simulink model "EV_Modeling_old"  (R2024b)
settings: Solver=FixedStepAuto  StartTime=0.0  StopTime=10382  FixedStep=0.1  RelTol=1e-3
values from neighbouring files (symbols this model uses):
  battery_SOC_SOC = battery_SOC(:,1)    [EV_Truck.m]    (also in simulink.m)
  battery_SOC_voltage = battery_SOC(:,2)    [EV_Truck.m]    (also in simulink.m)
  drag_coefficient_FV1 = table2array(drag_coefficient(:,3))    [simulink.m]
  drag_coefficient_FV2 = table2array(drag_coefficient(:,4))    [simulink.m]
  drag_coefficient_input = table2array(drag_coefficient(:,1))    [simulink.m]
  drag_coefficient_LV = table2array(drag_coefficient(:,2))    [simulink.m]
  electric_consumption_ressistancce = electric_consumption(:,2)    [EV_Truck.m]    (also in simulink.m)
  electric_consumption_voltage = electric_consumption(:,1)    [EV_Truck.m]    (also in simulink.m)
  motor_efficiency_efficiency = table2array(motor_efficiency(2:height(motor_efficiency),2:width(motor_efficiency)))    [EV_Truck.m]    (also in simulink.m)
  motor_efficiency_RPM = table2array(motor_efficiency(2:height(motor_efficiency),1))    [EV_Truck.m]    (also in simulink.m)
  motor_efficiency_torque = transpose(motor_efficiency_torque)    [EV_Truck.m]    (also in simulink.m)
  motor_RPM_torque = table2array(motor_torque(1:14,1))    [EV_Truck.m]    (also in simulink.m)
  motor_torque_RPM = table2array(motor_torque(1:14,2))    [EV_Truck.m]    (also in simulink.m)
undefined symbols (not defined in the file or in its folder): battery_builder_rtmsupport, battery_sli_rtmsupport, C1_mat, C2_mat, c_sqrt, DiscIntNeverNeededParam, dV0_mat, gcbh, n, Wc, Wm, x0
libraries: simulink x87, packLibrary_lib x30, nesl_utility x6, fl_lib x6, simulink_extras x3, mpcadaslib x2, slpidlib x1
(part 1 of 12)
settings Model: Creator=Administrator  LastModifiedBy=avees
settings SolverCC: AlgebraicLoopSolver=TrustRegion
settings DataIOCC: ExternalInput=EV_ModelingScenario.getElement('Input')  LoadExternalInput=on
settings DebuggingCC: UnconnectedInputMsg=warning  UnconnectedOutputMsg=warning  UnconnectedLineMsg=warning
settings ModelReferenceCC: EnableRefExpFcnMdlSchedulingChecks=on
settings RTWCC: GPUComputeCapability=3.5  DLArmComputeVersion=19.05

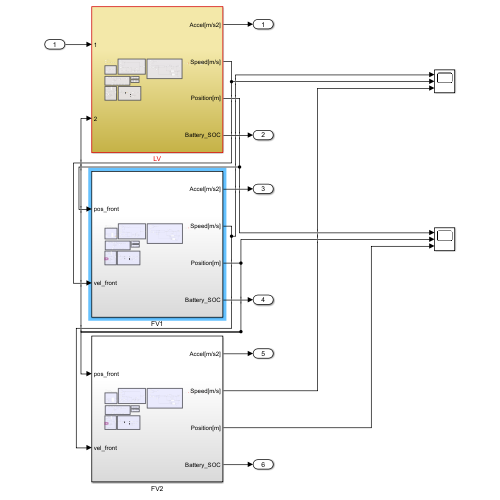
[thumbnail: Simulink's stored preview of the top-level diagram]
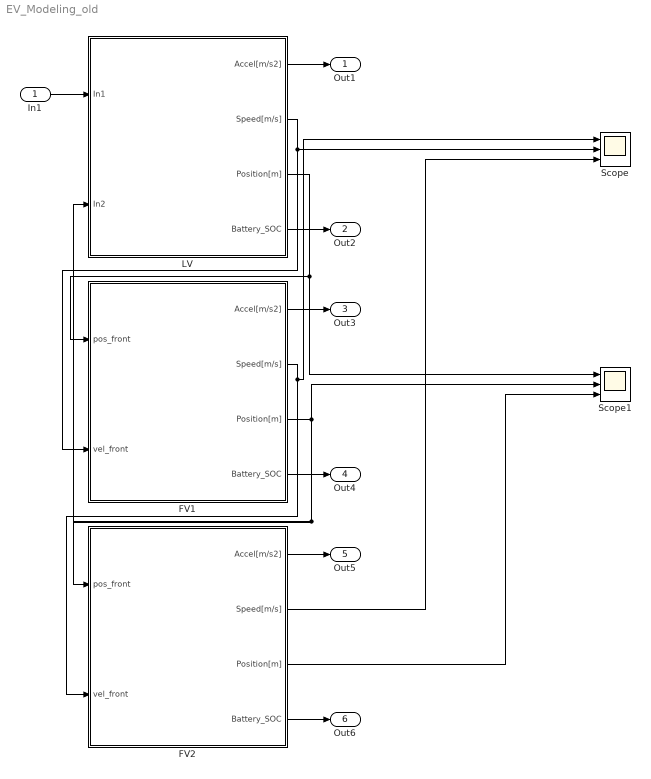
== system EV_Modeling_old ==
  In1 : Inport
  FV1 : Subsystem
  FV2 : Subsystem
  LV : Subsystem
  Scope : Scope  NumInputPorts=3
  Scope1 : Scope  NumInputPorts=3
  Out1 : Outport
  Out2 : Outport  Port=2
  Out3 : Outport  Port=3
  Out4 : Outport  Port=4
  Out5 : Outport  Port=5
  Out6 : Outport  Port=6
  wires:
  In1/1 -> LV/1(In1)
  LV/3(Position[m]) -> Scope1/1, FV1/1(pos_front)
  LV/2(Speed[m/s]) -> FV1/2(vel_front), Scope/2
  FV1/2(Speed[m/s]) -> FV2/2(vel_front), Scope/1
  FV1/3(Position[m]) -> LV/2(In2), FV2/1(pos_front), Scope1/2
  LV/1(Accel[m/s2]) -> Out1/1
  LV/4(Battery_SOC) -> Out2/1
  FV1/1(Accel[m/s2]) -> Out3/1
  FV1/4(Battery_SOC) -> Out4/1
  FV2/1(Accel[m/s2]) -> Out5/1
  FV2/2(Speed[m/s]) -> Scope/3
  FV2/3(Position[m]) -> Scope1/3
  FV2/4(Battery_SOC) -> Out6/1

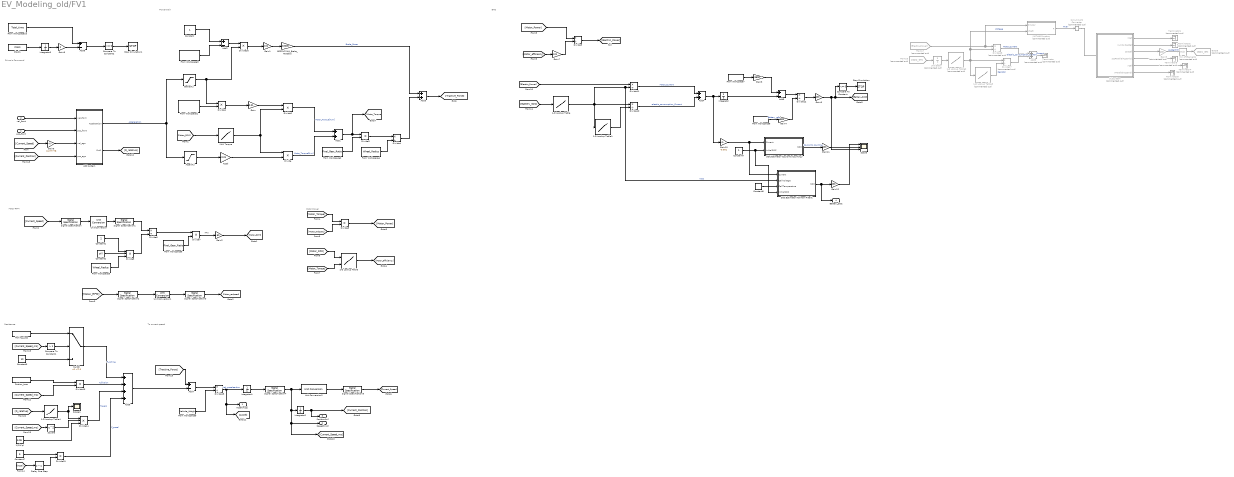
== system EV_Modeling_old/FV1 ==
  note: BMS
  note: To current speed
  note: Motor Power
  note: Power train
  note: Driver's Command
  note: RPS
  note: Motor RPM
  note: Resistance
  pos_front : Inport
  vel_front : Inport  Port=2
  1-D Lookup Table : Lookup_n-D  NumberOfTableDimensions=1  BreakpointsForDimension1=battery_SOC_SOC  Table=battery_SOC_voltage  InternalRulePriority=Speed  RndMeth=Simplest
  1-D Lookup Table1 : Lookup_n-D  NumberOfTableDimensions=1  BreakpointsForDimension1=electric_consumption_voltage  Table=electric_consumption_ressistancce  InternalRulePriority=Speed  RndMeth=Simplest
  1-D Lookup Table2 : Lookup_n-D  Commented=on  NumberOfTableDimensions=1  BreakpointsForDimension1=battery_SOC_SOC  Table=battery_SOC_voltage  InternalRulePriority=Speed  RndMeth=Simplest
  1-D Lookup Table3 : Lookup_n-D  Commented=on  NumberOfTableDimensions=1  BreakpointsForDimension1=electric_consumption_voltage  Table=electric_consumption_ressistancce  InternalRulePriority=Speed  RndMeth=Simplest
  1-D Lookup Table4 : Lookup_n-D  NumberOfTableDimensions=1  BreakpointsForDimension1=drag_coefficient_input  Table=drag_coefficient_FV1  InternalRulePriority=Speed  RndMeth=Simplest
  1/2(A*p) : Constant  Value=5.06
  2-D Lookup Table : Lookup_n-D  BreakpointsForDimension1=motor_efficiency_RPM  BreakpointsForDimension2=motor_efficiency_torque  Table=motor_efficiency_efficiency  InternalRulePriority=Speed  RndMeth=Simplest
      settings: InputPortMap=u0,u1
  ACC system : Subsystem
  Accel : Gain  Gain=0.01
  Accel[%] : Saturate  UpperLimit=100  LowerLimit=0
  Add1 : Sum
  Add{2,5,7..8} (4 alike) : Sum  Inputs=+-
  Add3 : Sum
  Add4 : Sum
  Add6 : Sum  Inputs=++++
  Add9 : Sum  Commented=on
  BPP[%]*MAX_Brake_Force[N] : Gain  Gain=10000
  Brake[%] : Saturate  UpperLimit=0  LowerLimit=-100
  Clock1 : simulink_extras/Flip Flops/Clock  period=2
  Compare To Constant : simulink/Logic and Bit Operations/Compare To Constant  relop=<=  const=0  OutDataTypeStr=boolean
  Compare To Constant1 : simulink/Logic and Bit Operations/Compare To Constant  relop=>  const=1  OutDataTypeStr=boolean
  Compare To Constant2 : simulink/Logic and Bit Operations/Compare To Constant  relop=<=  const=0  OutDataTypeStr=boolean
  Constant : Constant
  Constant1 : Constant  Value=2
  Constant2 : Constant  Value=pi()
  Constant3 : Constant  Value=10
  Constant4 : Constant
  Constant5 : Constant  Value=298.15
  Constant7 : Constant  Value=5
  Delay One Step : Delay  DelayLength=1
  Divide{,1..3,7..8,13,16,19} (9 alike) : Product  Inputs=**
  Divide{4,6,9..12,15} (7 alike) : Product  Inputs=*/
  Divide14 : Product  Inputs=***
  Divide17 : Product  Commented=on  Inputs=*/
  Divide18 : Product  Commented=on  Inputs=*/
  Divide5 : Product  Inputs=***
  Friction_Loss : FromWorkspace  VariableName=Resistance_friction
  From Workspace1 : FromWorkspace  VariableName=Regenerative_percent
  From Workspace10 : FromWorkspace  VariableName=Total_time
  From Workspace2 : FromWorkspace  VariableName=Final_Gear_Ratio
  From Workspace3 : FromWorkspace  VariableName=Regenerative_percent
  From Workspace4 : FromWorkspace  VariableName=Wheel_Radius
  From Workspace5 : FromWorkspace  VariableName=Wheel_Radius
  From Workspace6 : FromWorkspace  VariableName=Final_Gear_Ratio
  From Workspace7 : FromWorkspace  VariableName=Battery_Capacity
  From Workspace8 : FromWorkspace  VariableName=Battery_Capacity
  From Workspace9 : FromWorkspace  VariableName=Vehicle_Weight
  From16 : From  Commented=on  GotoTag=SOC_GT
  From17 : From  Commented=on  GotoTag=Electric_Power
  Gain : Gain  Gain=0.01
  Gain1 : Gain  Gain=0.01
  Gain10 : Gain  Gain=-0.001
  Gain11 : Gain  Gain=100
  Gain12 : Gain  Gain=100
  Gain2 : Gain  Gain=60
  Gain3 : Gain  Gain=3600
  Gain4 : Gain  Gain=3600
  Gain5 : Gain  Gain=100
  Gain6 : Gain  Gain=0.277778
  Gain7 : Gain  Gain=0.01
  Gain8 : Gain  Gain=2
  Gain9 : Gain  Commented=on  Gain=100
  Goto8 : Goto  Commented=on  GotoTag=SOC_GT
  Integrator{,1..3} (4 alike) : Integrator
  MATLAB Function : MATLAB Function  Commented=on  TreatAsAtomicUnit=on
  MAX Torque : Lookup_n-D  NumberOfTableDimensions=1  BreakpointsForDimension1=motor_RPM_torque  Table=motor_torque_RPM  InternalRulePriority=Speed  RndMeth=Simplest
  Min of Elements : MinMax  Commented=on
  Rolling_Loss : FromWorkspace  VariableName=Resistance_rolling
  SOC Estimator (Coulomb Counting) : Subsystem  AncestorBlock=|  LoadFcn=battery_sli_rtmsupport( 'loadfcn', gcbh );  TreatAsAtomicUnit=on  mask(SOC Estimator (Coulomb Counting)){CurrentInputPartition=on, AH=625, Ts=-1}
      | batt_sl_lib/Estimators/SOC Estimator
      | (Coulomb Counting)
      mask prompts: CurrentInputPartition "physmod:battery:library:comments:control:BatteryEstimators:SpecifyCurrentInputAsCellCurrents_MP"; AH "physmod:battery:library:comments:control:BatteryEstimators:CellCapacityAH_MP"; Ts "physmod:battery:library:comments:control:BatteryEstimators:SampleTime1ForInherited_MP"
      mask help: physmod:battery:library:comments:control:BatteryEstimators:CoulombCounting_MD
      mask init:
      | battery.mask.initializeCoulombCounter(AH,Ts);
      | battery.mask.initializeCurrentInputPartition([gcb '/For Each'],CurrentInputPartition);
      settings: CopyFcn=battery_sli_rtmsupport( 'copyfcn', gcbh );  DeleteFcn=battery_sli_rtmsupport( 'deletefcn', gcbh );  ModelCloseFcn=battery_sli_rtmsupport( 'modelclosefcn', gcbh );  PostSaveFcn=battery_sli_rtmsupport( 'postsavefcn', gcbh );  PreCopyFcn=battery_sli_rtmsupport( 'precopyfcn', gcbh );  OpenFcn=battery_sli_rtmsupport( 'openfcn', gcbh );  CloseFcn=battery_sli_rtmsupport( 'closefcn', gcbh );  PreDeleteFcn=battery_sli_rtmsupport( 'predeletefcn', gcbh );
      settings: LibrarySourceBlock=|
      | batt_sl_lib/Estimators/SOC Estimator
      | (Coulomb Counting)
      mask Help: web(nesl_help(gcbh))
      mask TypeOptions Ts: Integrator/Ts
      mask DialogControl CurrentInputPartition Prompt: 전류 입력을 셀 전류로 지정
      mask DialogControl AH Prompt: 셀 용량, AH(A*Hr)
      mask DialogControl Ts Prompt: 샘플 시간(상속된 경우 -1)
  SOC Estimator (Kalman Filter)1 : Subsystem  AncestorBlock=|  LoadFcn=battery_sli_rtmsupport( 'loadfcn', gcbh );  TreatAsAtomicUnit=on  mask(SOC Estimator (Kalman Filter)){CurrentInputPartition=on, filterType=Extended Kalman filter, alpha=1, beta=2, kappa=0, Q=|, Q_2RC=|, R=0.1, P0=[1e-5 0; 0 1], P0_2RC=[1e-5 0 0; 0 1 0;0 0 1], Ts=1, chargeDynamics=One time-constant dynamics, SOC_vec=[0.0, 0.01, 0.02, 0.03, 0.04, 0.05, 0.06, 0.07, 0.08, 0.09, 0.1, 0.11, 0.12, 0.13, 0.14, 0.15, 0.16, 0.17, 0.18, 0.19, 0.2, 0.21, 0.22, 0.23, 0.24, 0.25, 0.26, 0.27, 0.28, 0.29, 0.3, 0.31, 0.32, 0.33, 0.34, 0.35, 0.36, 0.37, 0.38, 0.39, 0.4, 0.41, 0.42, 0.43, 0.44, 0.45, 0.46, 0.47, 0.48, 0.49, 0.5, 0.51, 0.52, 0.53, 0.54, 0.55, 0.56, 0.57, 0.58, 0.59, 0.6, 0.61, 0.62, 0.63, 0.64, 0.65, 0.66, 0.67, 0.68, 0.69, 0.7, 0.71, 0.72, 0.73, 0.74, 0.75, 0.76, 0.77, 0.78, 0.79, 0.8, 0.81, 0.82, 0.83, 0.84, 0.85, 0.86, 0.87, 0.88, 0.89, 0.9, 0.91, 0.92, 0.93, 0.94, 0.95, 0.96, 0.97, 0.98, 0.99, 1.0], T_vec=298.15, R0_mat=[0.03361043165467626; 0.030818920863309354; 0.028460575539568343; 0.026631654676258994; 0.024979208633093528; 0.023567410071942445; 0.02242834532374101; 0.021465755395683454; 0.020583381294964027; 0.01987748201438849; 0.019187625899280573; 0.018529856115107914; 0.017904172661870502; 0.017310575539568343; 0.01671697841726619; 0.01615546762589928; 0.01562604316546763; 0.01522496402877698; 0.01482388489208633; 0.014438848920863306; 0.014053812949640289; 0.013716906474820146; 0.013524388489208634; 0.013347913669064747; 0.013251654676258993; 0.013235611510791367; 0.013235611510791367; 0.013251654676258993; 0.013267697841726617; 0.013283741007194243; 0.013315827338129497; 0.01338; 0.013444172661870504; 0.013508345323741008; 0.013604604316546762; 0.013716906474820146; 0.01384525179856115; 0.013973597122302159; 0.014101942446043163; 0.014230287769784172; 0.01435863309352518; 0.014486978417266186; 0.014615323741007194; 0.014727625899280576; 0.014839928057553955; 0.014936187050359713; 0.015048489208633092; 0.0151768345323741; 0.015289136690647482; 0.015417482014388488; 0.015529784172661869; 0.015658129496402877; 0.015898776978417267; 0.016043165467625898; 0.01609129496402878; 0.016139424460431654; 0.016251726618705036; 0.016396115107913667; 0.016524460431654675; 0.016636762589928057; 0.01673302158273381; 0.01682928057553957; 0.016925539568345326; 0.017021798561151078; 0.01710201438848921; 0.017198273381294964; 0.017278489208633094; 0.01735870503597122; 0.017454964028776977; 0.01753517985611511; 0.017631438848920863; 0.01772769784172662; 0.017872086330935254; 0.018048561151079136; 0.018225035971223023; 0.018417553956834535; 0.01862611510791367; 0.01885071942446043; 0.01905928057553957; 0.019283884892086333; 0.019492446043165468; 0.019701007194244603; 0.019909568345323737; 0.020102086330935253; 0.020230431654676258; 0.020358776978417266; 0.020455035971223022; 0.020535251798561152; 0.020615467625899282; 0.020679640287769786; 0.020759856115107913; 0.020824028776978417; 0.020791942446043165; 0.02072776978417266; 0.02072776978417266; 0.02066359712230216; 0.020567338129496404; 0.020535251798561152; 0.019765179856115107; 0.019476402877697842; 0.015273093525179856], R1_mat=[0.00465251798561151; 0.003850359712230215; 0.004171223021582734; 0.002566906474820144; 0.003689928057553957; 0.002887769784172662; 0.002727338129496403;0.00465251798561151; 0.003850359712230215; 0.004171223021582734; 0.002566906474820144; 0.003689928057553957; 0.002887769784172662; 0.002727338129496403;0.00465251798561151; 0.003850359712230215; 0.004171223021582734; 0.002566906474820144; 0.003689928057553957; 0.002887769784172662; 0.002727338129496403;0.00465251798561151; 0.003850359712230215; 0.004171223021582734; 0.002566906474820144; 0.003689928057553957; 0.002887769784172662; 0.002727338129496403;0.00465251798561151; 0.003850359712230215; 0.004171223021582734; 0.002566906474820144; 0.003689928057553957; 0.002887769784172662; 0.002727338129496403;0.00465251798561151; 0.003850359712230215; 0.004171223021582734; 0.002566906474820144; 0.003689928057553957; 0.002887769784172662; 0.002727338129496403;0.00465251798561151; 0.003850359712230215; 0.004171223021582734; 0.002566906474820144; 0.003689928057553957; 0.002887769784172662; 0.002727338129496403;0.00465251798561151; 0.003850359712230215; 0.004171223021582734; 0.002566906474820144; 0.003689928057553957; 0.002887769784172662; 0.002727338129496403;0.00465251798561151; 0.003850359712230215; 0.004171223021582734; 0.002566906474820144; 0.003689928057553957; 0.002887769784172662; 0.002727338129496403;0.00465251798561151; 0.003850359712230215; 0.004171223021582734; 0.002566906474820144; 0.003689928057553957; 0.002887769784172662; 0.002727338129496403;0.00465251798561151; 0.003850359712230215; 0.004171223021582734; 0.002566906474820144; 0.003689928057553957; 0.002887769784172662; 0.002727338129496403;0.00465251798561151; 0.003850359712230215; 0.004171223021582734; 0.002566906474820144; 0.003689928057553957; 0.002887769784172662; 0.002727338129496403;0.00465251798561151; 0.003850359712230215; 0.004171223021582734; 0.002566906474820144; 0.003689928057553957; 0.002887769784172662; 0.002727338129496403;0.00465251798561151; 0.003850359712230215; 0.004171223021582734; 0.002566906474820144; 0.003689928057553957; 0.002887769784172662; 0.002727338129496403;0.003689928057553957; 0.002887769784172662; 0.002727338129496403], tau1_mat=[36.0; 44.99999999999999; 104.99999999999999; 29.000000000000004; 77.0; 33.0; 39.00000000000001;36.0; 44.99999999999999; 104.99999999999999; 29.000000000000004; 77.0; 33.0; 39.00000000000001;36.0; 44.99999999999999; 104.99999999999999; 29.000000000000004; 77.0; 33.0; 39.00000000000001;36.0; 44.99999999999999; 104.99999999999999; 29.000000000000004; 77.0; 33.0; 39.00000000000001;36.0; 44.99999999999999; 104.99999999999999; 29.000000000000004; 77.0; 33.0; 39.00000000000001;36.0; 44.99999999999999; 104.99999999999999; 29.000000000000004; 77.0; 33.0; 39.00000000000001;36.0; 44.99999999999999; 104.99999999999999; 29.000000000000004; 77.0; 33.0; 39.00000000000001;36.0; 44.99999999999999; 104.99999999999999; 29.000000000000004; 77.0; 33.0; 39.00000000000001;36.0; 44.99999999999999; 104.99999999999999; 29.000000000000004; 77.0; 33.0; 39.00000000000001;36.0; 44.99999999999999; 104.99999999999999; 29.000000000000004; 77.0; 33.0; 39.00000000000001;36.0; 44.99999999999999; 104.99999999999999; 29.000000000000004; 77.0; 33.0; 39.00000000000001;36.0; 44.99999999999999; 104.99999999999999; 29.000000000000004; 77.0; 33.0; 39.00000000000001;36.0; 44.99999999999999; 104.99999999999999; 29.000000000000004; 77.0; 33.0; 39.00000000000001;36.0; 44.99999999999999; 104.99999999999999; 29.000000000000004; 77.0; 33.0; 39.00000000000001;77.0; 33.0; 39.00000000000001], R2_mat=[.0109, .0029, .0013; .0069, .0024, .0012; .0047, .0026, .0013; .0034, .0016, .001; .0033, .0023, .0014; .0033, .0018, .0011; .0028, .0017, .0011], tau2_mat=[20, 36, 39; 31, 45, 39; 109, 105, 61; 36, 29, 26; 59, 77, 67; 40, 33, 29; 25, 39, 33], V0_mat=[707.44966; 709.74656; 712.0434600000001; 714.33813; 716.63503; 718.93193; 721.22883; 723.52573; 725.82263; 728.1173; 730.4141999999999; 732.7111; 735.0079999999999; 737.3049; 739.5995700000001; 741.89647; 744.1933700000001; 746.49027; 748.7871700000001; 751.08407; 753.37874; 755.6756399999999; 757.97254; 760.2694399999999; 762.56634; 764.8632399999999; 767.15791; 769.4548100000001; 771.75171; 774.04861; 776.34551; 778.64018; 780.93708; 783.23398; 785.53088; 787.82778; 790.12468; 792.41935; 794.7162500000001; 797.01315; 799.31005; 801.60695; 803.90385; 806.19852; 808.49542; 810.79232; 813.08922; 815.38612; 817.68079; 819.9776899999999; 822.2745900000001; 824.57149; 827.42143; 829.81199; 831.7833099999999; 833.75686; 836.05376; 838.33728; 840.60073; 842.7393000000001; 844.86895; 846.92501; 848.98107; 850.9903; 852.9950699999999; 855.00207; 857.00684; 859.01161; 861.01861; 863.02338; 865.01923; 867.0931300000001; 869.30752; 871.67801; 874.0507299999999; 876.4167600000001; 878.78279; 881.15774; 883.49032; 885.81398; 888.13764; 890.46353; 892.7135999999999; 894.7228299999999; 896.3351200000001; 897.9496399999999; 899.3277800000001; 900.63902; 901.77409; 902.8824; 903.99071; 905.0967899999999; 906.07576; 907.05919; 908.3525900000001; 910.10091; 911.85592; 914.1015299999999; 916.77753; 922.77846; 929.53313], AH=27}
      | batt_sl_lib/Estimators/SOC Estimator
      | (Kalman Filter)
      mask Q=|
      | [1e-6 0;
      | 0 1e-6]
      mask Q_2RC=|
      | [1e-6 0 0;
      | 0 1e-6 0; 0 0 1e-6]
      mask prompts: CurrentInputPartition "physmod:battery:library:comments:control:BatteryEstimators:SpecifyCurrentInputAsCellCurrents_MP"; filterType "physmod:battery:library:comments:control:BatteryEstimators:FilterType_MP"; alpha "physmod:battery:library:comments:control:BatteryEstimators:Alpha_MP"; beta "physmod:battery:library:comments:control:BatteryEstimators:Beta_MP"; kappa "physmod:battery:library:comments:control:BatteryEstimators:Kappa_MP"; Q "physmod:battery:library:comments:control:BatteryEstimators:CovarianceOfTheProcessNoiseQ_MP"; Q_2RC "physmod:battery:library:comments:control:BatteryEstimators:CovarianceOfTheProcessNoiseQ_MP"; R "physmod:battery:library:comments:control:BatteryEstimators:CovarianceOfTheMeasurementNoiseR_MP"; P0 "physmod:battery:library:comments:control:BatteryEstimators:InitialStateErrorCovarianceP0_MP"; P0_2RC "physmod:battery:library:comments:control:BatteryEstimators:InitialStateErrorCovarianceP0_MP"; Ts "physmod:battery:library:comments:control:BatteryEstimators:SampleTime1ForInherited_MP"; chargeDynamics "physmod:battery:library:comments:control:BatteryEstimators:ChargeDynamics_MP"; SOC_vec "physmod:battery:library:comments:control:BatteryEstimators:VectorOfStateofchargeValuesSOC_MP"; T_vec "physmod:battery:library:comments:control:BatteryEstimators:VectorOfTemperaturesT_MP"; R0_mat "physmod:battery:library:comments:control:BatteryEstimators:TerminalResistanceR0SOCT_MP"; R1_mat "physmod:battery:library:comments:control:BatteryEstimators:FirstPolarizationResistanceR1SOCT_MP"; tau1_mat "physmod:battery:library:comments:control:BatteryEstimators:FirstTimeConstantTau1SOCT_MP"; R2_mat "physmod:battery:library:comments:control:BatteryEstimators:SecondPolarizationResistanceR2SOCT_MP"; tau2_mat "physmod:battery:library:comments:control:BatteryEstimators:SecondTimeConstantTau2SOCT_MP"; V0_mat "physmod:battery:library:comments:control:BatteryEstimators:NoloadVoltageV0SOCT_MP"; AH "physmod:battery:library:comments:control:BatteryEstimators:CellCapacityAH_MP"
      mask help: physmod:battery:library:comments:control:BatteryEstimators:SOCEstimatorKalmanFilter_MD
      mask init:
      | [C1_mat,C2_mat,dV0_mat,m,n,Wm,Wc,c_sqrt] = battery.mask.initializeKalmanFilter(filterType,chargeDynamics,tau1_mat,R1_mat,tau2_mat,R2_mat,V0_mat,SOC_vec,T_vec,P0,P0_2RC,R,Q,Q_2RC,alpha,beta,kappa,Ts,AH,R0_mat);%#ok
      | battery.mask.initializeCurrentInputPartition([gcb '/For Each'],CurrentInputPartition);
      settings: CopyFcn=battery_sli_rtmsupport( 'copyfcn', gcbh );  DeleteFcn=battery_sli_rtmsupport( 'deletefcn', gcbh );  ModelCloseFcn=battery_sli_rtmsupport( 'modelclosefcn', gcbh );  PostSaveFcn=battery_sli_rtmsupport( 'postsavefcn', gcbh );  PreCopyFcn=battery_sli_rtmsupport( 'precopyfcn', gcbh );  OpenFcn=battery_sli_rtmsupport( 'openfcn', gcbh );  CloseFcn=battery_sli_rtmsupport( 'closefcn', gcbh );  PreDeleteFcn=battery_sli_rtmsupport( 'predeletefcn', gcbh );
      settings: LibrarySourceBlock=|
      | batt_sl_lib/Estimators/SOC Estimator
      | (Kalman Filter)
      mask Help: web(nesl_help(gcbh))
      mask TypeOptions filterType: Kalman Filter/filterType
      mask Callback filterType: battery.mask.callbackPopupKalmanFilter(gcb);
      mask TypeOptions chargeDynamics: Kalman Filter/chargeDynamics
      mask Callback chargeDynamics: battery.mask.callbackPopupChargeDynamics(gcb);
      mask DialogControl Container6 Prompt: physmod:battery:library:comments:control:BatteryEstimators:tab_Main
      mask DialogControl CurrentInputPartition Prompt: 전류 입력을 셀 전류로 지정
      mask DialogControl filterType Prompt: 필터 유형
      mask DialogControl alpha Prompt: 알파
      mask DialogControl beta Prompt: 베타
      mask DialogControl kappa Prompt: 카파
      mask DialogControl Q Prompt: 공정 잡음의 공분산, Q
      mask DialogControl Q_2RC Prompt: 공정 잡음의 공분산, Q
      mask DialogControl R Prompt: 측정 잡음의 공분산, R
      mask DialogControl P0 Prompt: 초기 상태 오차 공분산, P0
      mask DialogControl P0_2RC Prompt: 초기 상태 오차 공분산, P0
      mask DialogControl Ts Prompt: 샘플 시간(상속된 경우 -1)
      mask DialogControl Container4 Prompt: physmod:battery:library:comments:control:BatteryEstimators:tab_SystemModel
      mask DialogControl chargeDynamics Prompt: 충전 동특성
      mask DialogControl SOC_vec Prompt: 충전 상태 값으로 구성된 벡터, SOC(-)
      mask DialogControl T_vec Prompt: 온도로 구성된 벡터, T
      mask DialogControl R0_mat Prompt: 단자 저항, R0(SOC,T), (ohm)
      mask DialogControl R1_mat Prompt: 1차 분극 저항, R1(SOC,T), (ohm)
      mask DialogControl tau1_mat Prompt: 1차 시정수, tau1(SOC,T), (s)
      mask DialogControl R2_mat Prompt: 2차 분극 저항, R2(SOC,T), (ohm)
      mask DialogControl tau2_mat Prompt: 2차 시정수, tau2(SOC,T), (s)
      mask DialogControl V0_mat Prompt: 무부하 전압, V0(SOC,T), (V)
      mask DialogControl AH Prompt: 셀 용량, AH(A*Hr)
  Scope : Scope  NumInputPorts=3
  Scope1 : Scope
  Signal Specification : SignalSpecification  Unit=km/hr
  Signal Specification1 : SignalSpecification  Unit=m/s
  Signal Specification2 : SignalSpecification  Unit=rpm
  Signal Specification3 : SignalSpecification  Unit=rad/s
  Signal Specification4 : SignalSpecification  Unit=m/s
  Signal Specification5 : SignalSpecification  Unit=km/hr
  Simulink-PS Converter : nesl_utility/Simulink-PS Converter  Commented=on  PhysicalDomain=network_engine_domain  SubClassName=ps_input  LeftPortType=input  RightPortType=output  PseudoPeriodic=off  Frequencies=[]  NoiseDistribution=none  NoiseParameters=[]  Unit=Ohm  AffineConversion=off  FilteringAndDerivatives=provide  SimscapeFilterOrder=1  InputFilterTimeConstant=0.001  UdotUserProvided=0
  Square : Math  Operator=square
  Stop Simulation : Stop
  Stop Simulation1 : Stop
  Subsystem : Subsystem  Commented=on
  Switch : Switch  Criteria=u2 ~= 0  SaturateOnIntegerOverflow=off  InputSameDT=off
  Terminator{,1..5} (6 alike) : Terminator  Commented=on
  Unit Conversion : UnitConversion
  Unit Conversion1 : UnitConversion
  Unit Conversion2 : UnitConversion
  Unit Delay : UnitDelay  Commented=on  SampleTime=-1  HasFrameUpgradeWarning=on
  Accel[m/s2] : Outport
  Speed[m/s] : Outport  Port=2
  Position[m] : Outport  Port=3
  Battery_SOC : Outport  Port=4
  wires:
  Signal Specification3/1 -> [Motor_radpsec]
  From Workspace5/1 -> Divide5/3
  Divide1/1 -> Gain/1
  [Motor_RPM] -> Signal Specification2/1
  Gain11/1 -> Scope/2
  Divide/1 -> Add1/2  "Motor_Torque[N.m]"
  Gain12/1 -> Scope/1
  Divide7/1 -> Gain2/1
  Gain5/1 -> Scope/3, [Battery_SOC], Compare To Constant/1
  Constant4/1 -> SOC Estimator (Kalman Filter)1/4(InitialSOC), SOC Estimator (Coulomb Counting)/2(InitialSOC)
  Signal Specification5/1 -> [Current_Speed]
  Brake[%]/1 -> Divide16/2, Divide1/1
  From Workspace8/1 -> Gain4/1  "Battery_cap"
  Accel/1 -> Divide/2
  1-D Lookup Table1/1 -> Divide10/2
  Divide12/1 -> Gain5/1
  From17/1 -> MATLAB Function/1(Pmotor), Divide18/1
  1-D Lookup Table2/1 -> 1-D Lookup Table3/1, Divide17/1, MATLAB Function/2(Vbatt), Divide18/2  "Voltage"
  [Current_Speed] -> Gain6/1
  MAX Torque/1 -> Divide2/2, Divide/1
  Divide17/1 -> Add9/2  "electric_consumption_Current"
  Subsystem/2(numCyclesCell) -> Terminator2/1
  From Workspace1/1 -> Divide1/2
  Min of Elements/1 -> Goto8/1
  Divide4/1 -> Add3/2
  From16/1 -> Unit Delay/1
  Constant1/1 -> Divide5/1
  [Motor_Torque] -> Divide8/1
  From Workspace9/1 -> Divide15/2
  Subsystem/1(iCell) -> Terminator1/1
  Divide11/1 -> Add4/1  "Motor_Current"
  Divide18/1 -> Add9/1  "Motor_Current"
  1-D Lookup Table/1 -> Divide10/1, SOC Estimator (Kalman Filter)1/2(CellVoltage), Divide11/2, 1-D Lookup Table1/1  "Vsoc"
  Divide16/1 -> Gain1/1
  1-D Lookup Table3/1 -> Divide17/2  "Resistor"
  From Workspace3/1 -> Add2/2
  Integrator2/1 -> [Current_Position], Position[m]/1
  From Workspace4/1 -> Divide4/2
  Add5/1 -> Divide12/1
  Add1/1 -> Divide3/1, [Motor_Torque]
  Add2/1 -> Divide16/1
  Divide8/1 -> [Motor_Power]
  [Electric_Power] -> Divide11/1
  From Workspace10/1 -> Add8/1
  [Motor_Torque] -> 2-D Lookup Table/2
  Unit Delay/1 -> 1-D Lookup Table2/1
  Signal Specification/1 -> Unit Conversion/1
  Subsystem/6(vParallelAssembly) -> Terminator5/1
  Divide6/1 -> Divide7/1
  Add7/1 -> Divide15/1
  Divide3/1 -> Divide4/1
  Subsystem/3(socCell) -> Gain9/1
  [Motor_RPM] -> 2-D Lookup Table/1
  [Motor_Power] -> Divide9/1
  Accel[%]/1 -> Accel/1
  Gain7/1 -> Divide9/2
  Constant/1 -> Add2/1
  Gain3/1 -> Add5/1
  Add4/1 -> Gain10/1, Integrator/1
  Gain4/1 -> Divide12/2
  Divide5/1 -> Divide6/2
  Integrator/1 -> Add5/2
  [Current_Speed] -> Signal Specification/1
  2-D Lookup Table/1 -> [Motor_efficiency]
  BPP[%]*MAX_Brake_Force[N]/1 -> Add3/1  "Brake_Force"
  Clock1/1 -> Integrator3/1
  Divide9/1 -> [Electric_Power]
  Signal Specification4/1 -> [Current_Speed_ms], Speed[m/s]/1, Integrator2/1, Unit Conversion2/1
  [Tractive_Force] -> Add7/1
  [Battery_SOC] -> 1-D Lookup Table/1
  Add3/1 -> [Tractive_Force]
  Divide15/1 -> [Accel], Accel[m/s2]/1, Integrator1/1  "Veh_acceleartion"
  Add8/1 -> Compare To Constant2/1
  MATLAB Function/1(R) -> Simulink-PS Converter/1  "Rvar"
  [Motor_RPM] -> MAX Torque/1
  Gain9/1 -> Min of Elements/1  "socCelllllll"
  Compare To Constant/1 -> Stop Simulation/1
  Gain8/1 -> Add8/2
  Gain2/1 -> [Motor_RPM]
  Subsystem/5(vCell) -> Terminator4/1
  Integrator3/1 -> Gain8/1
  Divide10/1 -> Add4/2  "electric_consumption_Current"
  Unit Conversion2/1 -> Signal Specification5/1
  Unit Conversion1/1 -> Signal Specification3/1
  Constant2/1 -> Divide5/2
  ACC system/1(Acceleration) -> Accel[%]/1, Brake[%]/1  "Acceleration"
  Unit Conversion/1 -> Signal Specification1/1
  [Motor_efficiency] -> Gain7/1
  Signal Specification1/1 -> Divide6/1
  Divide2/1 -> Add1/1  "Motor_Torque[N.m]"
  Compare To Constant2/1 -> Stop Simulation1/1
  [Motor_radpsec] -> Divide8/2
  Gain1/1 -> BPP[%]*MAX_Brake_Force[N]/1
  Add9/1 -> Terminator/1  "Current"
  From Workspace2/1 -> Divide3/2
  From Workspace7/1 -> Gain3/1
  From Workspace6/1 -> Divide7/2
  Subsystem/4(socParallelAssembly) -> Terminator3/1
  Integrator1/1 -> Signal Specification4/1
  Signal Specification2/1 -> Unit Conversion1/1
  Gain/1 -> Divide2/1
  Constant5/1 -> SOC Estimator (Kalman Filter)1/3(CellTemperature)
  SOC Estimator (Coulomb Counting)/1(SOC) -> Gain11/1  "Coulomb counting"
  Gain10/1 -> SOC Estimator (Kalman Filter)1/1(Current), SOC Estimator (Coulomb Counting)/1(Current)
  SOC Estimator (Kalman Filter)1/1(SOC) -> Battery_SOC/1, Gain12/1
  [Current_Position] -> ACC system/4(pos_ego)
  vel_front/1 -> ACC system/1(vel_front)
  pos_front/1 -> ACC system/2(pos_front)
  Gain6/1 -> ACC system/3(vel_ego)
  [Current_Speed_ms] -> Square/1
  [Current_Speed_ms] -> Divide13/2
  Constant7/1 -> Divide19/1
  Divide14/1 -> Add6/3  "F_aero"
  Delay One Step/1 -> Divide19/2
  [Current_Speed_ms] -> Compare To Constant1/1
  [Accel] -> Delay One Step/1
  1-D Lookup Table4/1 -> Scope1/1, Divide14/1
  Friction_Loss/1 -> Divide13/1
  Constant3/1 -> Switch/3
  1/2(A*p)/1 -> Divide14/3
  Square/1 -> Divide14/2
  Rolling_Loss/1 -> Switch/1
  Divide19/1 -> Add6/4  "F_accel"
  Switch/1 -> Add6/1  "F_rolling"
  Compare To Constant1/1 -> Switch/2
  Divide13/1 -> Add6/2  "F_friction"
  Add6/1 -> Add7/2
  [D_relative] -> 1-D Lookup Table4/1
  ACC system/2(Out1) -> [D_relative]
  connections:
  Simulink-PS Converter/RConn1 -- Subsystem/LConn1
